simulink model "cantx_2X"  (R2022b)
settings: configuration reference "SLDD_CFG" (kept outside this file)
libraries: user_lib x8, simulink x3
settings Model: DataDictionary=cantx_2X.sldd  Creator=Castiel  LastModifiedBy=Castiel
settings ConfigSetRef: SourceName=SLDD_CFG

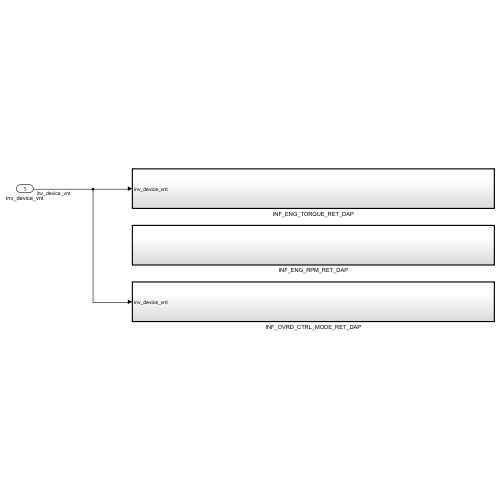
[thumbnail: Simulink's stored preview of the top-level diagram]
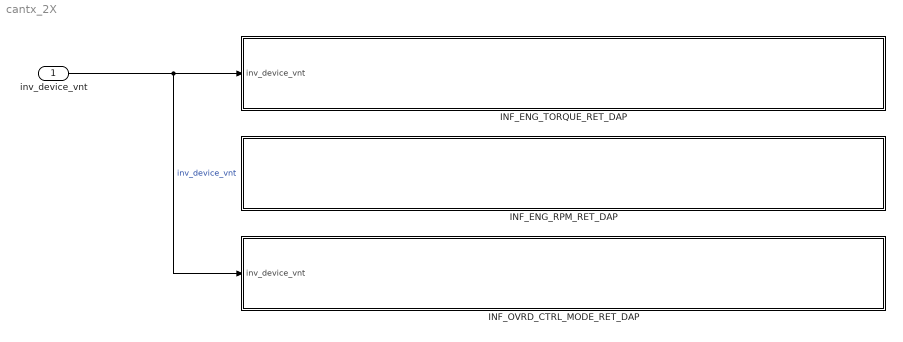
== system cantx_2X ==
  inv_device_vnt : Inport
  INF_ENG_RPM_RET_DAP : Subsystem  TreatAsAtomicUnit=on
      settings: RTWSystemCode=Nonreusable function
  INF_ENG_TORQUE_RET_DAP : Subsystem  TreatAsAtomicUnit=on
      settings: RTWSystemCode=Nonreusable function
  INF_OVRD_CTRL_MODE_RET_DAP : Subsystem  TreatAsAtomicUnit=on
      settings: RTWSystemCode=Nonreusable function
  wires:
  inv_device_vnt/1 -> INF_ENG_TORQUE_RET_DAP/1(inv_device_vnt), INF_OVRD_CTRL_MODE_RET_DAP/1(inv_device_vnt)  "inv_device_vnt"

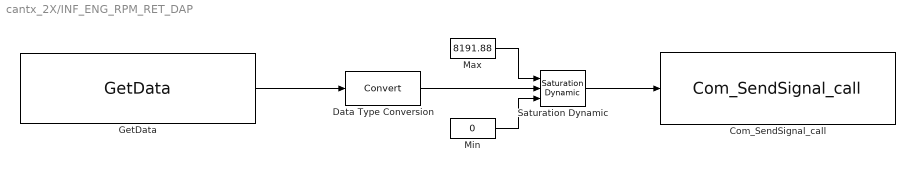
== system cantx_2X/INF_ENG_RPM_RET_DAP ==
  Com_SendSignal_call : user_lib/Com_SendSignal_call  signalId=id3
      settings: SourceProductName=User Defined for IFLayer
  Data Type Conversion : DataTypeConversion  ConvertRealWorld=Stored Integer (SI)  SaturateOnIntegerOverflow=off  RndMeth=Floor
  GetData : user_lib/GetData  interface=INF_ENG_RPM_RET_DAP  signalType=UW
      settings: SourceProductName=User Defined for IFLayer
  Max : Constant  Value=8191.88  OutDataTypeStr=Inherit: Inherit via back propagation
  Min : Constant  Value=0  OutDataTypeStr=Inherit: Inherit via back propagation
  Saturation Dynamic : simulink/Discontinuities/Saturation Dynamic  OutMin=[]  OutMax=[]  OutDataTypeStr=Inherit: Same as second input  OutDataType=fixdt(1, 16)  OutScaling=2^-10  DoSatur=off
  wires:
  Saturation Dynamic/1 -> Com_SendSignal_call/1
  Min/1 -> Saturation Dynamic/3
  Max/1 -> Saturation Dynamic/1
  GetData/1 -> Data Type Conversion/1
  Data Type Conversion/1 -> Saturation Dynamic/2

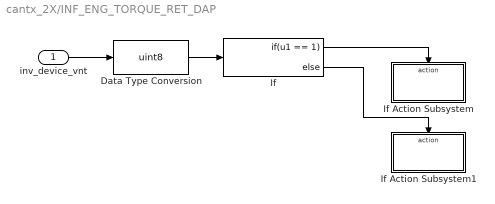
== system cantx_2X/INF_ENG_TORQUE_RET_DAP ==
  inv_device_vnt : Inport
  Data Type Conversion : DataTypeConversion  OutDataTypeStr=uint8  SaturateOnIntegerOverflow=off  RndMeth=Floor
  If : If  IfExpression=u1 == 1
  If Action Subsystem : Subsystem  TreatAsAtomicUnit=on
  If Action Subsystem1 : Subsystem  TreatAsAtomicUnit=on
  wires:
  Data Type Conversion/1 -> If/1
  inv_device_vnt/1 -> Data Type Conversion/1
  If/1 -> If Action Subsystem/Action
  If/2 -> If Action Subsystem1/Action

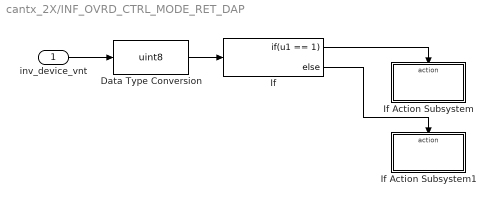
== system cantx_2X/INF_OVRD_CTRL_MODE_RET_DAP ==
  inv_device_vnt : Inport
  Data Type Conversion : DataTypeConversion  OutDataTypeStr=uint8  SaturateOnIntegerOverflow=off  RndMeth=Floor
  If : If  IfExpression=u1 == 1
  If Action Subsystem : Subsystem  TreatAsAtomicUnit=on
  If Action Subsystem1 : Subsystem  TreatAsAtomicUnit=on
  wires:
  Data Type Conversion/1 -> If/1
  inv_device_vnt/1 -> Data Type Conversion/1
  If/1 -> If Action Subsystem/Action
  If/2 -> If Action Subsystem1/Action

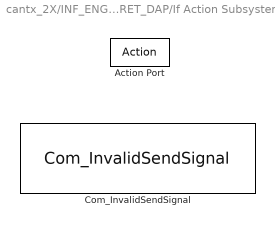
== system cantx_2X/INF_ENG_TORQUE_RET_DAP/If Action Subsystem ==
  Action Port : ActionPort
  Com_InvalidSendSignal : user_lib/Com_InvalidSendSignal  signalId=id1
      settings: SourceProductName=User Defined for IFLayer

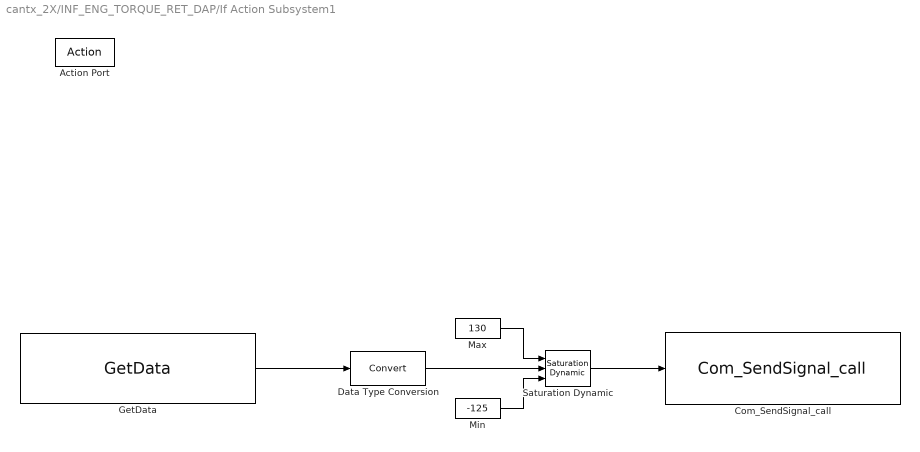
== system cantx_2X/INF_ENG_TORQUE_RET_DAP/If Action Subsystem1 ==
  Action Port : ActionPort
  Com_SendSignal_call : user_lib/Com_SendSignal_call  signalId=id1
      settings: SourceProductName=User Defined for IFLayer
  Data Type Conversion : DataTypeConversion  ConvertRealWorld=Stored Integer (SI)  SaturateOnIntegerOverflow=off  RndMeth=Floor
  GetData : user_lib/GetData  interface=INF_ENG_TORQUE_RET_DAP  signalType=SB
      settings: SourceProductName=User Defined for IFLayer
  Max : Constant  Value=130  OutDataTypeStr=Inherit: Inherit via back propagation
  Min : Constant  Value=-125  OutDataTypeStr=Inherit: Inherit via back propagation
  Saturation Dynamic : simulink/Discontinuities/Saturation Dynamic  OutMin=[]  OutMax=[]  OutDataTypeStr=Inherit: Same as second input  OutDataType=fixdt(1, 16)  OutScaling=2^-10  DoSatur=off
  wires:
  Saturation Dynamic/1 -> Com_SendSignal_call/1
  GetData/1 -> Data Type Conversion/1
  Min/1 -> Saturation Dynamic/3
  Data Type Conversion/1 -> Saturation Dynamic/2
  Max/1 -> Saturation Dynamic/1

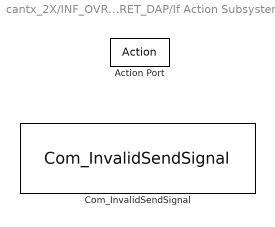
== system cantx_2X/INF_OVRD_CTRL_MODE_RET_DAP/If Action Subsystem ==
  Action Port : ActionPort
  Com_InvalidSendSignal : user_lib/Com_InvalidSendSignal  signalId=id5
      settings: SourceProductName=User Defined for IFLayer

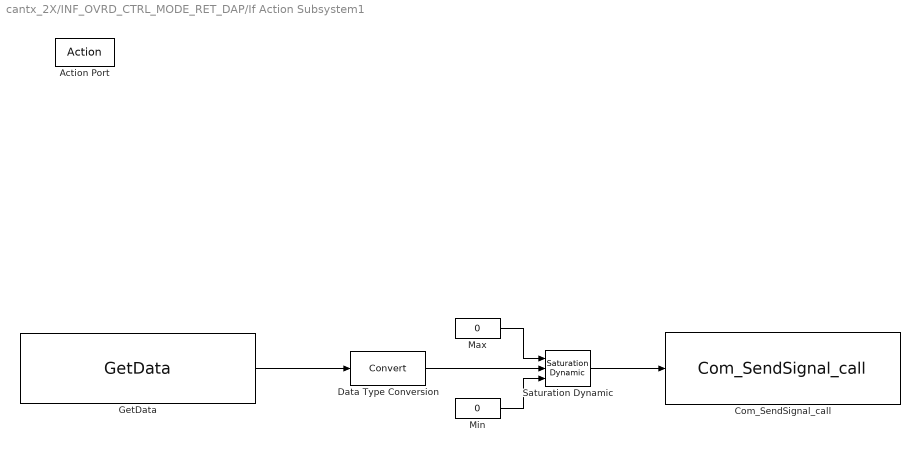
== system cantx_2X/INF_OVRD_CTRL_MODE_RET_DAP/If Action Subsystem1 ==
  Action Port : ActionPort
  Com_SendSignal_call : user_lib/Com_SendSignal_call  signalId=id5
      settings: SourceProductName=User Defined for IFLayer
  Data Type Conversion : DataTypeConversion  ConvertRealWorld=Stored Integer (SI)  SaturateOnIntegerOverflow=off  RndMeth=Floor
  GetData : user_lib/GetData  interface=INF_OVRD_CTRL_MODE_RET_DAP  signalType=UB
      settings: SourceProductName=User Defined for IFLayer
  Max : Constant  Value=0  OutDataTypeStr=Inherit: Inherit via back propagation
  Min : Constant  Value=0  OutDataTypeStr=Inherit: Inherit via back propagation
  Saturation Dynamic : simulink/Discontinuities/Saturation Dynamic  OutMin=[]  OutMax=[]  OutDataTypeStr=Inherit: Same as second input  OutDataType=fixdt(1, 16)  OutScaling=2^-10  DoSatur=off
  wires:
  Saturation Dynamic/1 -> Com_SendSignal_call/1
  GetData/1 -> Data Type Conversion/1
  Min/1 -> Saturation Dynamic/3
  Data Type Conversion/1 -> Saturation Dynamic/2
  Max/1 -> Saturation Dynamic/1
